simulink model "Adder"  (R2018a)
settings: Solver=VariableStepAuto  StartTime=0.0  StopTime=10.0  RelTol=1e-3
settings Model: Creator=midog  LastModifiedBy=midog

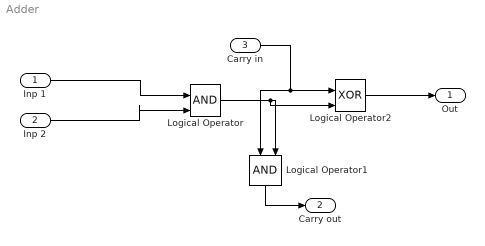
== system Adder ==
  Inp 1 : Inport
  Inp 2 : Inport  Port=2
  Carry in : Inport  Port=3
  Logical Operator : Logic  IconShape=distinctive  AllPortsSameDT=off  OutDataTypeStr=boolean
  Logical Operator1 : Logic  IconShape=distinctive  AllPortsSameDT=off  OutDataTypeStr=boolean
  Logical Operator2 : Logic  Operator=XOR  IconShape=distinctive  AllPortsSameDT=off  OutDataTypeStr=boolean
  Out : Outport
  Carry out : Outport  Port=2
  wires:
  Logical Operator1/1 -> Carry out/1
  Logical Operator/1 -> Logical Operator2/2, Logical Operator1/2
  Carry in/1 -> Logical Operator1/1, Logical Operator2/1
  Inp 2/1 -> Logical Operator/2
  Inp 1/1 -> Logical Operator/1
  Logical Operator2/1 -> Out/1
